simulink model "exam2021"  (R2021b)
settings: Solver=VariableStepAuto  StartTime=0.0  StopTime=100  RelTol=1e-3
settings Model: Creator=rohan  LastModifiedBy=rohan

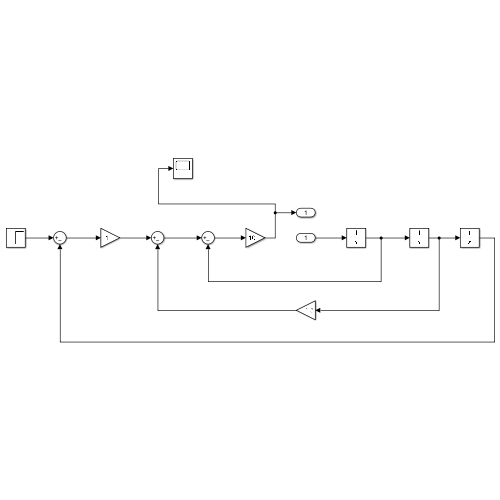
[thumbnail: Simulink's stored preview of the top-level diagram]
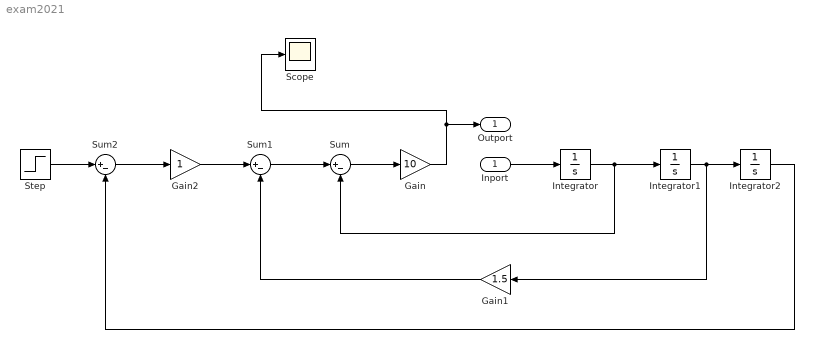
== system exam2021 ==
  Inport : Inport
  Gain : Gain  Gain=10
  Gain1 : Gain  Gain=1.5
  Gain2 : Gain
  Integrator : Integrator
  Integrator1 : Integrator
  Integrator2 : Integrator
  Scope : Scope
  Step : Step  After=1.50615  SampleTime=0
  Sum : Sum  Inputs=|+-
  Sum1 : Sum  Inputs=|+-
  Sum2 : Sum  Inputs=|+-
  Outport : Outport
  wires:
  Gain/1 -> Outport/1, Scope/1
  Inport/1 -> Integrator/1
  Sum/1 -> Gain/1
  Integrator/1 -> Integrator1/1, Sum/2
  Integrator1/1 -> Gain1/1, Integrator2/1
  Sum1/1 -> Sum/1
  Gain1/1 -> Sum1/2
  Gain2/1 -> Sum1/1
  Sum2/1 -> Gain2/1
  Integrator2/1 -> Sum2/2
  Step/1 -> Sum2/1
